simulink library "fixpt_megmalib"  (Simulink 6.0)
settings: Solver=ode45  SolverMode=SingleTasking  StartTime=0.0  StopTime=10.0  RelTol=1e-3
undefined symbols (not defined in the file or in its folder): Bias1, Bias2, NumBits1, NumBits2, Slope1, Slope2
libraries: simulink x94, fixpt_megmaFuncBlkhidden1 x5, fixpt_megmalib x3
(part 2 of 3)

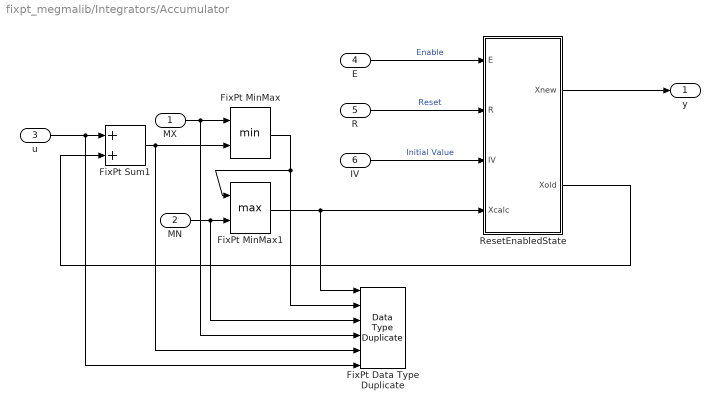
== system fixpt_megmalib/Integrators/Accumulator ==
  MX : Inport  LatchInput=off
  MN : Inport  Port=2  LatchInput=off
  u : Inport  Port=3  LatchInput=off
  E : Inport  Port=4  LatchInput=off
  R : Inport  Port=5  LatchInput=off
  IV : Inport  Port=6  LatchInput=off
  FixPt Data Type Duplicate : simulink/Signal Attributes/Data Type Duplicate  NumInputPorts=6
  FixPt MinMax : MinMax  Inputs=2  OutScaling=2^-10  ZeroCross=off
  FixPt MinMax1 : MinMax  Function=max  Inputs=2  OutScaling=2^-10  ZeroCross=off
  FixPt Sum1 : Sum  OutDataType=uint(4)  OutScaling=1  LockScale=on
  ResetEnabledState : Subsystem  PropExecContextAcrossSSBoundary=on
  y : Outport
  wires:
  ResetEnabledState/2(Xold) -> FixPt Sum1/2
  ResetEnabledState/1(Xnew) -> y/1
  IV/1 -> ResetEnabledState/3(IV)  "Initial Value"
  E/1 -> ResetEnabledState/1(E)  "Enable"
  R/1 -> ResetEnabledState/2(R)  "Reset"
  FixPt MinMax1/1 -> FixPt Data Type Duplicate/1, ResetEnabledState/4(Xcalc)
  MN/1 -> FixPt Data Type Duplicate/3, FixPt MinMax1/2
  FixPt MinMax/1 -> FixPt Data Type Duplicate/2, FixPt MinMax1/1
  MX/1 -> FixPt Data Type Duplicate/4, FixPt MinMax/1
  FixPt Sum1/1 -> FixPt Data Type Duplicate/5, FixPt MinMax/2
  u/1 -> FixPt Data Type Duplicate/6, FixPt Sum1/1

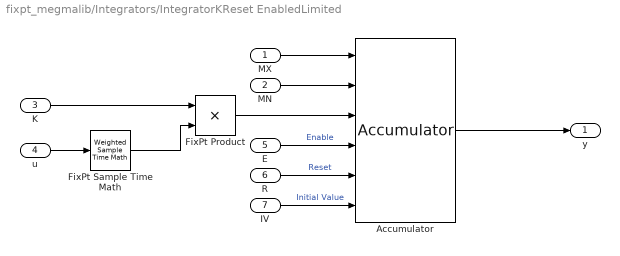
== system fixpt_megmalib/Integrators/IntegratorKReset EnabledLimited ==
  MX : Inport  LatchInput=off
  MN : Inport  Port=2  LatchInput=off
  K : Inport  Port=3  LatchInput=off
  u : Inport  Port=4  LatchInput=off
  E : Inport  Port=5  LatchInput=off
  R : Inport  Port=6  LatchInput=off
  IV : Inport  Port=7  LatchInput=off
  Accumulator : fixpt_megmalib/Integrators/Accumulator
  FixPt Product : Product  OutScaling=2^-10
  FixPt Sample Time Math : simulink/Math Operations/Weighted Sample Time Math  TsampMathOp=*  weightValue=1.0  TsampMathImp=Online Calculations  DoSatur=off
  y : Outport
  wires:
  Accumulator/1 -> y/1
  K/1 -> FixPt Product/1
  FixPt Sample Time Math/1 -> FixPt Product/2
  u/1 -> FixPt Sample Time Math/1
  FixPt Product/1 -> Accumulator/3
  MX/1 -> Accumulator/1
  MN/1 -> Accumulator/2
  R/1 -> Accumulator/5  "Reset"
  E/1 -> Accumulator/4  "Enable"
  IV/1 -> Accumulator/6  "Initial Value"

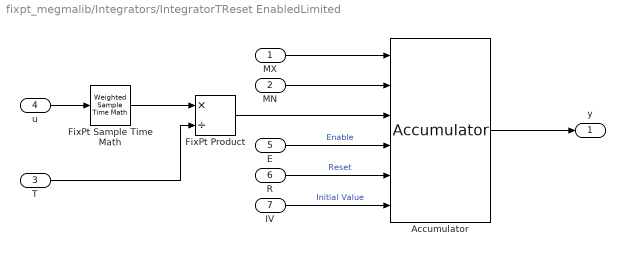
== system fixpt_megmalib/Integrators/IntegratorTReset EnabledLimited ==
  MX : Inport  LatchInput=off
  MN : Inport  Port=2  LatchInput=off
  T : Inport  Port=3  LatchInput=off
  u : Inport  Port=4  LatchInput=off
  E : Inport  Port=5  LatchInput=off
  R : Inport  Port=6  LatchInput=off
  IV : Inport  Port=7  LatchInput=off
  Accumulator : fixpt_megmalib/Integrators/Accumulator
  FixPt Product : Product  Inputs=*/  OutScaling=2^-10
  FixPt Sample Time Math : simulink/Math Operations/Weighted Sample Time Math  TsampMathOp=*  weightValue=1.0  TsampMathImp=Online Calculations  DoSatur=off
  y : Outport
  wires:
  Accumulator/1 -> y/1
  FixPt Product/1 -> Accumulator/3
  MX/1 -> Accumulator/1
  MN/1 -> Accumulator/2
  R/1 -> Accumulator/5  "Reset"
  E/1 -> Accumulator/4  "Enable"
  IV/1 -> Accumulator/6  "Initial Value"
  u/1 -> FixPt Sample Time Math/1
  FixPt Sample Time Math/1 -> FixPt Product/1
  T/1 -> FixPt Product/2

== system fixpt_megmalib/Low and Highpass/DigitalLowPass ResetEnabled ==
  m : Inport  LatchInput=off
  U : Inport  Port=2  LatchInput=off
  E : Inport  Port=3  LatchInput=off
  R : Inport  Port=4  LatchInput=off
  IV : Inport  Port=5  LatchInput=off
  Combine Terms1 : Sum  Description=\nAdd in CPU  OutDataType=sfix(32)  OutScaling=2^-24
  Difference Inputs : Sum  Description=\nAdd in CPU  Inputs=+-  OutDataType=BaseType  OutScaling=1
  FixPt Data Type Duplicate : simulink/Signal Attributes/Data Type Duplicate  NumInputPorts=6
  FixPt Product : Product  OutScaling=2^-10
  ResetEnabledState : Subsystem  PropExecContextAcrossSSBoundary=on
  y : Outport
  wires:
  m/1 -> FixPt Product/1
  Difference Inputs/1 -> FixPt Data Type Duplicate/4, FixPt Product/2
  U/1 -> FixPt Data Type Duplicate/5, Difference Inputs/1  "U(k)"
  ResetEnabledState/2(Xold) -> FixPt Data Type Duplicate/1, Difference Inputs/2, Combine Terms1/2  "Xold"
  ResetEnabledState/1(Xnew) -> y/1  "Xnew"
  E/1 -> ResetEnabledState/1(E)  "Enable"
  IV/1 -> FixPt Data Type Duplicate/6, ResetEnabledState/3(IV)  "Initial Value"
  R/1 -> ResetEnabledState/2(R)  "Reset"
  Combine Terms1/1 -> FixPt Data Type Duplicate/2, ResetEnabledState/4(Xcalc)  "Y(k)"
  FixPt Product/1 -> FixPt Data Type Duplicate/3, Combine Terms1/1

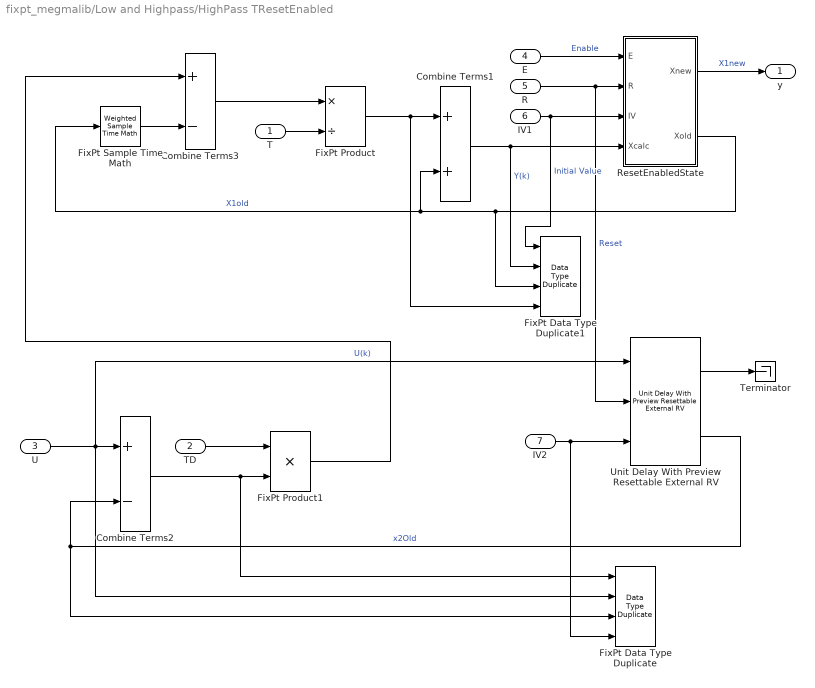
== system fixpt_megmalib/Low and Highpass/HighPass TResetEnabled ==
  T : Inport  LatchInput=off
  TD : Inport  Port=2  LatchInput=off
  U : Inport  Port=3  LatchInput=off
  E : Inport  Port=4  LatchInput=off
  R : Inport  Port=5  LatchInput=off
  IV1 : Inport  Port=6  LatchInput=off
  IV2 : Inport  Port=7  LatchInput=off
  Combine Terms1 : Sum  Description=\nAdd in CPU  OutDataType=sfix(32)  OutScaling=2^-24
  Combine Terms2 : Sum  Description=\nAdd in CPU  Inputs=+-  OutDataType=sfix(32)  OutScaling=2^-24
  Combine Terms3 : Sum  Description=\nAdd in CPU  Inputs=+-  OutDataType=sfix(32)  OutScaling=2^-24
  FixPt Data Type Duplicate : simulink/Signal Attributes/Data Type Duplicate  NumInputPorts=4
  FixPt Data Type Duplicate1 : simulink/Signal Attributes/Data Type Duplicate  NumInputPorts=4
  FixPt Product : Product  Inputs=*/  OutScaling=2^-10
  FixPt Product1 : Product  Inputs=**  OutScaling=2^-10
  FixPt Sample Time Math : simulink/Math Operations/Weighted Sample Time Math  TsampMathOp=*  weightValue=1.0  TsampMathImp=Online Calculations  DoSatur=off
  ResetEnabledState : Subsystem  PropExecContextAcrossSSBoundary=on
  Terminator : Terminator
  Unit Delay With Preview Resettable External RV : simulink/Additional Math & Discrete/Additional Discrete/Unit Delay With Preview Resettable External RV  vinit=0.0  tsamp=-1
  y : Outport
  wires:
  FixPt Product1/1 -> Combine Terms3/1
  FixPt Sample Time Math/1 -> Combine Terms3/2
  Combine Terms3/1 -> FixPt Product/1
  Combine Terms2/1 -> FixPt Data Type Duplicate/1, FixPt Product1/2
  TD/1 -> FixPt Product1/1
  Unit Delay With Preview Resettable External RV/2 -> FixPt Data Type Duplicate/3, Combine Terms2/2  "x2Old"
  ResetEnabledState/2(Xold) -> FixPt Data Type Duplicate1/3, FixPt Sample Time Math/1, Combine Terms1/2  "X1old"
  Combine Terms1/1 -> FixPt Data Type Duplicate1/2, ResetEnabledState/4(Xcalc)  "Y(k)"
  T/1 -> FixPt Product/2
  IV2/1 -> FixPt Data Type Duplicate/4, Unit Delay With Preview Resettable External RV/3
  FixPt Product/1 -> FixPt Data Type Duplicate1/4, Combine Terms1/1
  R/1 -> ResetEnabledState/2(R), Unit Delay With Preview Resettable External RV/2  "Reset"
  IV1/1 -> FixPt Data Type Duplicate1/1, ResetEnabledState/3(IV)  "Initial Value"
  E/1 -> ResetEnabledState/1(E)  "Enable"
  ResetEnabledState/1(Xnew) -> y/1  "X1new"
  U/1 -> FixPt Data Type Duplicate/2, Combine Terms2/1, Unit Delay With Preview Resettable External RV/1  "U(k)"
  Unit Delay With Preview Resettable External RV/1 -> Terminator/1

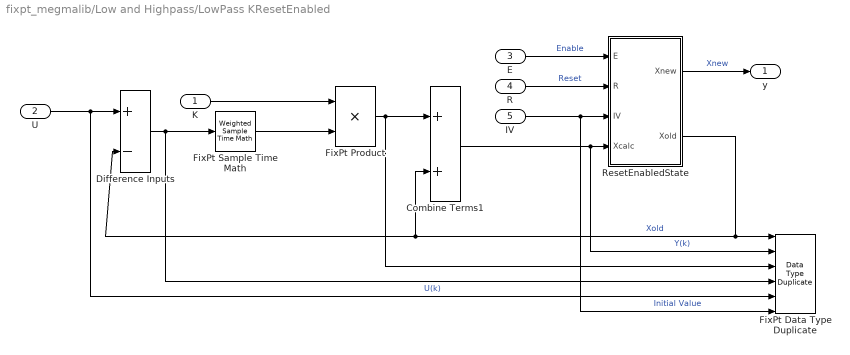
== system fixpt_megmalib/Low and Highpass/LowPass KResetEnabled ==
  K : Inport  LatchInput=off
  U : Inport  Port=2  LatchInput=off
  E : Inport  Port=3  LatchInput=off
  R : Inport  Port=4  LatchInput=off
  IV : Inport  Port=5  LatchInput=off
  Combine Terms1 : Sum  Description=\nAdd in CPU  OutDataType=sfix(32)  OutScaling=2^-24
  Difference Inputs : Sum  Description=\nAdd in CPU  Inputs=+-  OutDataType=BaseType  OutScaling=1
  FixPt Data Type Duplicate : simulink/Signal Attributes/Data Type Duplicate  NumInputPorts=6
  FixPt Product : Product  OutScaling=2^-10
  FixPt Sample Time Math : simulink/Math Operations/Weighted Sample Time Math  TsampMathOp=*  weightValue=1.0  TsampMathImp=Online Calculations  DoSatur=off
  ResetEnabledState : Subsystem  PropExecContextAcrossSSBoundary=on
  y : Outport
  wires:
  FixPt Sample Time Math/1 -> FixPt Product/2
  FixPt Product/1 -> Combine Terms1/1, FixPt Data Type Duplicate/3
  Combine Terms1/1 -> FixPt Data Type Duplicate/2, ResetEnabledState/4(Xcalc)  "Y(k)"
  R/1 -> ResetEnabledState/2(R)  "Reset"
  IV/1 -> FixPt Data Type Duplicate/6, ResetEnabledState/3(IV)  "Initial Value"
  E/1 -> ResetEnabledState/1(E)  "Enable"
  ResetEnabledState/1(Xnew) -> y/1  "Xnew"
  ResetEnabledState/2(Xold) -> Combine Terms1/2, Difference Inputs/2, FixPt Data Type Duplicate/1  "Xold"
  U/1 -> Difference Inputs/1, FixPt Data Type Duplicate/5  "U(k)"
  Difference Inputs/1 -> FixPt Data Type Duplicate/4, FixPt Sample Time Math/1
  K/1 -> FixPt Product/1

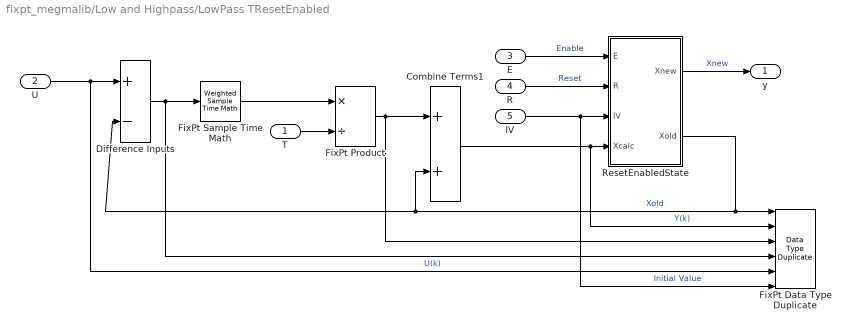
== system fixpt_megmalib/Low and Highpass/LowPass TResetEnabled ==
  T : Inport  LatchInput=off
  U : Inport  Port=2  LatchInput=off
  E : Inport  Port=3  LatchInput=off
  R : Inport  Port=4  LatchInput=off
  IV : Inport  Port=5  LatchInput=off
  Combine Terms1 : Sum  Description=\nAdd in CPU  OutDataType=sfix(32)  OutScaling=2^-24
  Difference Inputs : Sum  Description=\nAdd in CPU  Inputs=+-  OutDataType=BaseType  OutScaling=1
  FixPt Data Type Duplicate : simulink/Signal Attributes/Data Type Duplicate  NumInputPorts=6
  FixPt Product : Product  Inputs=*/  OutScaling=2^-10
  FixPt Sample Time Math : simulink/Math Operations/Weighted Sample Time Math  TsampMathOp=*  weightValue=1.0  TsampMathImp=Online Calculations  DoSatur=off
  ResetEnabledState : Subsystem  PropExecContextAcrossSSBoundary=on
  y : Outport
  wires:
  T/1 -> FixPt Product/2
  Difference Inputs/1 -> FixPt Sample Time Math/1, FixPt Data Type Duplicate/4
  U/1 -> FixPt Data Type Duplicate/5, Difference Inputs/1  "U(k)"
  ResetEnabledState/2(Xold) -> FixPt Data Type Duplicate/1, Difference Inputs/2, Combine Terms1/2  "Xold"
  ResetEnabledState/1(Xnew) -> y/1  "Xnew"
  E/1 -> ResetEnabledState/1(E)  "Enable"
  IV/1 -> FixPt Data Type Duplicate/6, ResetEnabledState/3(IV)  "Initial Value"
  R/1 -> ResetEnabledState/2(R)  "Reset"
  Combine Terms1/1 -> FixPt Data Type Duplicate/2, ResetEnabledState/4(Xcalc)  "Y(k)"
  FixPt Product/1 -> FixPt Data Type Duplicate/3, Combine Terms1/1
  FixPt Sample Time Math/1 -> FixPt Product/1

== system fixpt_megmalib/Mathematical Functions/Configurable Subsystem ==
  In1 : Inport  LatchInput=off
  Sine : fixpt_megmaFuncBlkhidden1/Sine  yData=[1 2 3]  xData=[1 2 3]  Recompute=Compute Always  Spacing='pow2'  Nptsmax=[]  ErrMax=0.01  RndMeth='floor'  yScale=2^-5  xScale=2^-5  yDt=sfix(16)  xDt=sfix(16)  xmax=2*pi  xmin=0
  Out1 : Outport
  wires:
  In1/1 -> Sine/1
  Sine/1 -> Out1/1

== system fixpt_megmalib/Mathematical Functions/Configurable Subsystem1 ==
  In1 : Inport  LatchInput=off
  Cosine : fixpt_megmaFuncBlkhidden1/Cosine  yData=[1 2 3]  xData=[1 2 3]  Recompute=Compute Always  yData_nonvisible=[1;0.999511758485136;0.998047510700099;0.995608686458002;0.992197667229329;0.987817783816472;0.982473313101255;0.976169473868635;0.968912421710645;0.960709243015562;0.951567948048172;0.941497463127881;0.930507621912314;0.918609155794918;0.905813683425936;0.892133699366994;0.877582561890373;0.86217447993488;0.845924499231068;0.828848487609326;0.810963119505218;0.792285859677179;0.772834946152472;0.752629372418066;0.731688868873821;0.71003388356608;0.687685562220505;0.664665727593633;0.640996858163325;0.616702066178912;0.591805075092477;0.566330196393309;0.54030230586814;0.513746819310368;0.486689667701963;0.459157271892304;0.431176516798666;0.402774725153557;0.373979630824533;0.344819351732545;0.315322362395269;0.28551746612222;0.255433766888812;0.225100640916817;0.194547707988987;0.163804802525833;0.132901944452825;0.101869309886441;0.0707372016677029;0.0395360197719658;0.00829623162385838;-0.0229516576536404;-0.0541771350269363;-0.0853497093472792;-0.116438941124852;-0.147414472252418;-0.178246055649492;-0.208903584798109;-0.239357123141322;-0.269576933315742;-0.299533506189574;-0.329197589677777;-0.358540217306233;-0.387532736497014;-0.416146836547142;-0.444354576273508;-0.47212841129696;-0.499441220938929;-0.526266334704305;-0.552577558324725;-0.578349199336833;-0.603556092170533;-0.628173622722739;-0.652177752392634;-0.675545041554953;-0.698252672448376;-0.720278471456692;-0.741600930760952;-0.762199229341495;-0.782053253309314;-0.801143615546934;-0.819451674639598;-0.836959553078294;-0.853650154716842;-0.869507181465984;-0.884515149208199;-0.898659402917676;-0.911926130970699;-0.924302378632464;-0.935776060707157;-0.946335973338945;-0.955971804952348;-0.964674146321316;-0.972434499757186;-0.979245287406521;-0.985099858650763;-0.989992496600445;-0.993918423677641;-0.996873806281181;-0.998855758530109;-0.999862345081687;-0.999892583021229;-0.9989464428219;-0.99702484837355;-0.994129676080546;-0.990263753029502;-0.98543085422867;-0.979635698921714;-0.972883945979446;-0.965182188374036;-0.956537946741083;-0.946959662035847;-0.936456687290796;-0.925039278482532;-0.912718584516998;-0.899506636342767;-0.88541633520302;-0.870461440037704;-0.85465655404816;-0.838017110437342;-0.820559357339561;-0.802300341954454;-0.783257893900684;-0.76345060780562;-0.742897825147999;-0.721619615371299;-0.699636756286272;-0.676970713781757;-0.653643620863612;-0.629678256042204;-0.605098021089583;-0.579926918188046;-0.554189526492417;-0.527910978128915;-0.501116933654064;-0.47383355699759;-0.446087489913793;-0.417905825966321;-0.38931608407177;-0.360346181627922;-0.331024407252887;-0.301379393161745;-0.271440087207671;-0.24123572461485;-0.21079579943078;-0.180150035725827;-0.149328358568183;-0.118360864802541;-0.0872777936610349;-0.0561094972351469;-0.0248864108374021;0.00636097671819611;0.0376021528879766;0.0688066111935807;0.0999438810110212;0.130983557324729;0.161895330417537;0.192649015467599;0.223214582023364;0.253562183327795;0.283662185463226;0.313485196288377;0.343002094139282;0.372184056266098;0.401002586978036;0.429429545468913;0.457437173296176;0.484998121486549;0.512085477241841;0.538672790218836;0.564734098357607;0.590243953233023;0.615177444904708;0.639510226241173;0.663218536694376;0.686279225501496;0.70866977429126;0.730368319072748;0.751353671585211;0.771605339988047;0.791103548870739;0.809829258563201;0.827764183727699;0.844890811214172;0.861192417161521;0.876653083328182;0.891257712636015;0.904992043912346;0.917842665815758;0.929797029932041;0.940843463027505;0.950971178447692;0.960170286650366;0.968431804862477;0.975747665851692;0.982110725803907;0.987514771299061;0.991954525378437;0.995425652697519;0.997924763759387;0.999449418224499;0.999998127293645]  xData_nonvisible=[0;0.03125;0.0625;0.09375;0.125;0.15625;0.1875;0.21875;0.25;0.28125;0.3125;0.34375;0.375;0.40625;0.4375;0.46875;0.5;0.53125;0.5625;0.59375;0.625;0.65625;0.6875;0.71875;0.75;0.78125;0.8125;0.84375;0.875;0.90625;0.9375;0.96875;1;1.03125;1.0625;1.09375;1.125;1.15625;1.1875;1.21875;1.25;1.28125;1.3125;1.34375;1.375;1.40625;1.4375;1.46875;1.5;1.53125;1.5625;1.59375;1.625;1.65625;1.6875;1.71875;1.75;1.78125;1.8125;1.84375;1.875;1.90625;1.9375;1.96875;2;2.03125;2.0625;2.09375;2.125;2.15625;2.1875;2.21875;2.25;2.28125;2.3125;2.34375;2.375;2.40625;2.4375;2.46875;2.5;2.53125;2.5625;2.59375;2.625;2.65625;2.6875;2.71875;2.75;2.78125;2.8125;2.84375;2.875;2.90625;2.9375;2.96875;3;3.03125;3.0625;3.09375;3.125;3.15625;3.1875;3.21875;3.25;3.28125;3.3125;3.34375;3.375;3.40625;3.4375;3.46875;3.5;3.53125;3.5625;3.59375;3.625;3.65625;3.6875;3.71875;3.75;3.78125;3.8125;3.84375;3.875;3.90625;3.9375;3.96875;4;4.03125;4.0625;4.09375;4.125;4.15625;4.1875;4.21875;4.25;4.28125;4.3125;4.34375;4.375;4.40625;4.4375;4.46875;4.5;4.53125;4.5625;4.59375;4.625;4.65625;4.6875;4.71875;4.75;4.78125;4.8125;4.84375;4.875;4.90625;4.9375;4.96875;5;5.03125;5.0625;5.09375;5.125;5.15625;5.1875;5.21875;5.25;5.28125;5.3125;5.34375;5.375;5.40625;5.4375;5.46875;5.5;5.53125;5.5625;5.59375;5.625;5.65625;5.6875;5.71875;5.75;5.78125;5.8125;5.84375;5.875;5.90625;5.9375;5.96875;6;6.03125;6.0625;6.09375;6.125;6.15625;6.1875;6.21875;6.25;6.28125]  Spacing_nonvisible='pow2'  Nptsmax_nonvisible=[]  ErrMax_nonvisible=0.01  RndMeth_nonvisible='floor'  yScale_nonvisible=2^-5  yDt_nonvisible=sfix(16)  xScale_nonvisible=2^-5  xDt_nonvisible=sfix(16)  xMax_nonvisible=2*pi  xMin_nonvisible=0  Spacing='pow2'  Nptsmax=[]  ErrMax=0.01  RndMeth='floor'  yScale=2^-5  xScale=2^-5  yDt=sfix(16)  xDt=sfix(16)  xmax=2*pi  xmin=0
  Out1 : Outport
  wires:
  In1/1 -> Cosine/1
  Cosine/1 -> Out1/1

== system fixpt_megmalib/Mathematical Functions/Configurable Subsystem2 ==
  In1 : Inport  LatchInput=off
  Tangent : fixpt_megmaFuncBlkhidden1/Tangent  yData=[1 2 3]  xData=[1 2 3]  Recompute=Compute Always  Spacing='pow2'  Nptsmax=[]  ErrMax=0.01  RndMeth='floor'  yScale=2^-5  xScale=2^-5  yDt=sfix(16)  xDt=sfix(16)  xmax=2*pi  xmin=0
  Out1 : Outport
  wires:
  In1/1 -> Tangent/1
  Tangent/1 -> Out1/1

== system fixpt_megmalib/Mathematical Functions/Configurable Subsystem3 ==
  In1 : Inport  LatchInput=off
  Exponent : fixpt_megmaFuncBlkhidden1/Exponent  yData=[1 2 3]  xData=[1 2 3]  Recompute=Compute Always  yData_nonvisible=[1;1.0317434074991;1.06449445891786;1.09828514030783;1.13314845306683;1.1691184461695;1.20623024942098;1.2445201077661;1.28402541668774;1.32478475872887;1.3668379411738;1.41022603492571;1.4549914146182;1.50117780000012;1.54883029863413;1.59799544995063;1.64872127070013;1.7010573018484;1.7550546569603;1.81076607211939;1.86824595743222;1.92755045016754;1.98873746958229;2.05186677348798;2.11700001661267;2.18420081081562;2.25353478721321;2.32506966027712;2.3988752939671;2.47502376996303;2.55358945806293;2.63464908881563;2.71828182845905;2.80456935623723;2.89359594417176;2.98544853936536;3.08021684891803;3.17799342753884;3.27887376793867;3.38295639409247;3.49034295746184;3.60113833627218;3.7154507379411;3.83339180475841;3.95507672292058;4.08062433502646;4.21015725614396;4.34380199356104;4.48168907033806;4.62395315278208;4.7707331819676;4.92217250943229;5.07841903718008;5.23962536212849;5.40594892514117;5.57755216479126;5.75460267600573;5.93727337374561;6.12574266188199;6.32019460743274;6.52081912033011;6.72781213889469;6.94137582119704;7.16171874249371;7.38905609893065;7.62360991771274;7.86560927394489;8.11529051435645;8.37289748812726;8.6386817850411;8.91290298119874;9.1958288925309;9.48773583635853;9.78890890125589;10.0996422254801;10.4202392842386;10.7510131860764;11.0922869786702;11.4443939643311;11.8076780255212;12.1824939607035;12.5692078308534;12.9681973169691;13.3798520889305;13.8045741860671;14.242778409807;14.6948927287889;15.1613586968345;15.6426318841882;16.1391823224464;16.6514949636101;17.1800701537093;17.7254241214616;18.2880894824436;18.8686157592649;19.4675699182552;20.0855369231877;20.7231203065787;21.3809427591233;22.0596467378412;22.7598950935267;23.4823717181174;24.227782212611;24.9968545761854;25.7903399171931;26.6090131867249;27.4536739354601;28.3251470945409;29.2242837812349;30.1519621301721;31.1090881509677;32.0965966130693;33.1154519586923;34.166649244734;35.2512151145885;36.3702088008095;37.524723159601;38.7158857381472;39.9448598758219;41.2128458403547;42.5210820000628;43.8708460332935;45.2634561762588;46.7002725104795;48.1826982910988;49.7121813173595;51.2902153465857;52.9183415530491;54.5981500331442;56.3312813583435;58.119428177448;59.9643368696996;61.8678092503679;63.8317043304791;65.8579401324037;67.9484955630781;70.1054123466879;72.3307970187014;74.6268229832009;76.9957326355201;79.4398395522613;81.9615307508321;84.563269020706;87.2475953286865;90.0171313005218;92.8745817812945;95.8227374770869;98.8644776805016;102.0027730827;105.240688674702;108.58138674079;112.02812994692;115.584284527188;119.253323571426;123.038830417177;126.944502149322;130.974153210819;135.13171912804;139.421260354375;143.846966235843;148.413159102577;153.124298490199;157.984985495187;162.999967268501;168.174141651845;173.512561961112;179.020441921657;184.703160760245;190.56626845863;196.615491173896;202.856736830865;209.296100892025;215.939872310614;222.794539672674;229.866797534079;237.163552958717;244.69193226422;252.459287981826;260.473206037167;268.741513159002;277.272284523134;286.073851638959;295.154810486372;304.524029910962;314.190660285694;324.164142447555;334.454216917865;345.070933415282;356.024660670779;367.326096554181;378.986278522156;391.016594397853;403.428793492735;416.234998081446;429.447715240934;443.079849065385;457.144713268909;471.656044188264;486.628014198347;502.075245553524;518.012824668342;534.45631685155]  xData_nonvisible=[0;0.03125;0.0625;0.09375;0.125;0.15625;0.1875;0.21875;0.25;0.28125;0.3125;0.34375;0.375;0.40625;0.4375;0.46875;0.5;0.53125;0.5625;0.59375;0.625;0.65625;0.6875;0.71875;0.75;0.78125;0.8125;0.84375;0.875;0.90625;0.9375;0.96875;1;1.03125;1.0625;1.09375;1.125;1.15625;1.1875;1.21875;1.25;1.28125;1.3125;1.34375;1.375;1.40625;1.4375;1.46875;1.5;1.53125;1.5625;1.59375;1.625;1.65625;1.6875;1.71875;1.75;1.78125;1.8125;1.84375;1.875;1.90625;1.9375;1.96875;2;2.03125;2.0625;2.09375;2.125;2.15625;2.1875;2.21875;2.25;2.28125;2.3125;2.34375;2.375;2.40625;2.4375;2.46875;2.5;2.53125;2.5625;2.59375;2.625;2.65625;2.6875;2.71875;2.75;2.78125;2.8125;2.84375;2.875;2.90625;2.9375;2.96875;3;3.03125;3.0625;3.09375;3.125;3.15625;3.1875;3.21875;3.25;3.28125;3.3125;3.34375;3.375;3.40625;3.4375;3.46875;3.5;3.53125;3.5625;3.59375;3.625;3.65625;3.6875;3.71875;3.75;3.78125;3.8125;3.84375;3.875;3.90625;3.9375;3.96875;4;4.03125;4.0625;4.09375;4.125;4.15625;4.1875;4.21875;4.25;4.28125;4.3125;4.34375;4.375;4.40625;4.4375;4.46875;4.5;4.53125;4.5625;4.59375;4.625;4.65625;4.6875;4.71875;4.75;4.78125;4.8125;4.84375;4.875;4.90625;4.9375;4.96875;5;5.03125;5.0625;5.09375;5.125;5.15625;5.1875;5.21875;5.25;5.28125;5.3125;5.34375;5.375;5.40625;5.4375;5.46875;5.5;5.53125;5.5625;5.59375;5.625;5.65625;5.6875;5.71875;5.75;5.78125;5.8125;5.84375;5.875;5.90625;5.9375;5.96875;6;6.03125;6.0625;6.09375;6.125;6.15625;6.1875;6.21875;6.25;6.28125]  Spacing_nonvisible='pow2'  Nptsmax_nonvisible=[]  ErrMax_nonvisible=0.01  RndMeth_nonvisible='floor'  yScale_nonvisible=2^-5  yDt_nonvisible=sfix(16)  xScale_nonvisible=2^-5  xDt_nonvisible=sfix(16)  xMax_nonvisible=2*pi  xMin_nonvisible=0  Spacing='pow2'  Nptsmax=[]  ErrMax=0.01  RndMeth='floor'  yScale=2^-5  xScale=2^-5  yDt=sfix(16)  xDt=sfix(16)  xmax=2*pi  xmin=0
  Out1 : Outport
  wires:
  In1/1 -> Exponent/1
  Exponent/1 -> Out1/1

== system fixpt_megmalib/Mathematical Functions/Configurable Subsystem4 ==
  In1 : Inport  LatchInput=off
  Sqrt : fixpt_megmaFuncBlkhidden1/Sqrt  yData=[1 2 3]  xData=[1 2 3]  Recompute=Compute Always  Spacing='pow2'  Nptsmax=[]  ErrMax=0.01  RndMeth='floor'  yScale=2^-5  xScale=2^-5  yDt=sfix(16)  xDt=sfix(16)  xmax=2*pi  xmin=0
  Out1 : Outport
  wires:
  In1/1 -> Sqrt/1
  Sqrt/1 -> Out1/1

== system fixpt_megmalib/Memory Blocks/DeltaOneStep ==
  note: IV
  U : Inport  LatchInput=off
  R : Inport  Port=2  LatchInput=off
  R1 : Inport  Port=3  LatchInput=off
  Data Type Duplicate : simulink/Signal Attributes/Data Type Duplicate  NumInputPorts=4
  Delay Input1 : UnitDelay  Description=\nStore in Global RAM  SampleTime=-1
  Difference Inputs1 : Sum  Description=\nAdd in CPU  Inputs=+-  OutDataType=BaseType  OutScaling=1
  Switch : Switch  Criteria=u2 ~= 0
  Y : Outport  InitialOutput=0
  wires:
  U/1 -> Data Type Duplicate/2, Difference Inputs1/1, Delay Input1/1  "U(k)"
  R/1 -> Switch/2
  R1/1 -> Data Type Duplicate/4, Switch/1
  Delay Input1/1 -> Switch/3  "U(k-1)"
  Difference Inputs1/1 -> Data Type Duplicate/1, Y/1  "( U(k) - U(k-1) )"
  Switch/1 -> Data Type Duplicate/3, Difference Inputs1/2

== system fixpt_megmalib/Memory Blocks/DifferenceQuotient ==
  u : Inport  LatchInput=off
  R : Inport  Port=2  LatchInput=off
  IV : Inport  Port=3  LatchInput=off
  DeltaOneStep : fixpt_megmalib/Memory Blocks/DeltaOneStep
  Sample Time Divide : simulink/Math Operations/Weighted Sample Time Math  TsampMathOp=/  weightValue=1  TsampMathImp=Online Calculations  DoSatur=off
  Y : Outport  InitialOutput=0
  wires:
  Sample Time Divide/1 -> Y/1
  DeltaOneStep/1 -> Sample Time Divide/1
  u/1 -> DeltaOneStep/1
  R/1 -> DeltaOneStep/2
  IV/1 -> DeltaOneStep/3

== system fixpt_megmalib/Memory Blocks/EdgeBi ==
  note: x
  U(k) : Inport  LatchInput=off
  R : Inport  Port=2  LatchInput=off
  IV : Inport  Port=3  LatchInput=off
  Data Type Duplicate : simulink/Signal Attributes/Data Type Duplicate  NumInputPorts=3
  Delay Input1 : UnitDelay  Description=\nStore in Global RAM  SampleTime=-1
  FixPt Relational Operator : RelationalOperator  Operator=~=  LogicOutDataTypeMode=Specify via dialog
  Switch : Switch  Criteria=u2 ~= 0
  Y : Outport  InitialOutput=0
  wires:
  U(k)/1 -> Delay Input1/1, FixPt Relational Operator/1
  FixPt Relational Operator/1 -> Y/1  "Edge"
  R/1 -> Switch/2
  IV/1 -> Data Type Duplicate/2, Switch/1
  Delay Input1/1 -> Data Type Duplicate/3, Switch/3  "U(k-1)"
  Switch/1 -> Data Type Duplicate/1, FixPt Relational Operator/2

== system fixpt_megmalib/Memory Blocks/EdgeFalling ==
  note: x
  U(k) : Inport  LatchInput=off
  R : Inport  Port=2  LatchInput=off
  IV : Inport  Port=3  LatchInput=off
  Data Type Duplicate : simulink/Signal Attributes/Data Type Duplicate  NumInputPorts=3
  Delay Input1 : UnitDelay  Description=\nStore in Global RAM  SampleTime=-1
  Logical Operator : Logic  Operator=NOT  Inputs=1  AllPortsSameDT=off  OutDataTypeMode=Specify via dialog
  Logical Operator1 : Logic  AllPortsSameDT=off  OutDataTypeMode=Specify via dialog
  Switch : Switch  Criteria=u2 ~= 0
  Y : Outport  InitialOutput=0
  wires:
  Delay Input1/1 -> Data Type Duplicate/2, Switch/3  "U(k-1)"
  IV/1 -> Data Type Duplicate/3, Switch/1
  R/1 -> Switch/2
  Logical Operator1/1 -> Y/1  "Edge"
  U(k)/1 -> Delay Input1/1, Logical Operator/1
  Switch/1 -> Data Type Duplicate/1, Logical Operator1/2
  Logical Operator/1 -> Logical Operator1/1

== system fixpt_megmalib/Memory Blocks/EdgeRising ==
  note: x
  U(k) : Inport  LatchInput=off
  R : Inport  Port=2  LatchInput=off
  IV : Inport  Port=3  LatchInput=off
  Data Type Duplicate : simulink/Signal Attributes/Data Type Duplicate  NumInputPorts=3
  Delay Input1 : UnitDelay  Description=\nStore in Global RAM  SampleTime=-1
  Logical Operator : Logic  Operator=NOT  Inputs=1  AllPortsSameDT=off  OutDataTypeMode=Specify via dialog
  Logical Operator1 : Logic  AllPortsSameDT=off  OutDataTypeMode=Specify via dialog
  Switch : Switch  Criteria=u2 ~= 0
  Y : Outport  InitialOutput=0
  wires:
  U(k)/1 -> Delay Input1/1, Logical Operator1/1
  Logical Operator1/1 -> Y/1  "Edge"
  R/1 -> Switch/2
  IV/1 -> Data Type Duplicate/2, Switch/1
  Delay Input1/1 -> Data Type Duplicate/3, Switch/3  "U(k-1)"
  Switch/1 -> Data Type Duplicate/1, Logical Operator/1
  Logical Operator/1 -> Logical Operator1/2

== system fixpt_megmalib/Memory Blocks/RSFlipFlop ==
  S : Inport  LatchInput=off
  R : Inport  Port=2  LatchInput=off
  Constant : Constant  OutDataTypeMode=boolean
  FixPt Data Type Duplicate1 : simulink/Signal Attributes/Data Type Duplicate  NumInputPorts=5
  FixPt Switch1 : Switch  Threshold=1
  FixPt Switch3 : Switch  Threshold=1
  FixPt Unit Delay1 : UnitDelay  X0=0.0  SampleTime=-1
  Ground : Ground
  Logical Operator : Logic  Operator=NOT  Inputs=1  AllPortsSameDT=off
  Q : Outport  InitialOutput=0
  !Q : Outport  Port=2  InitialOutput=1
  wires:
  Logical Operator/1 -> !Q/1
  Ground/1 -> FixPt Data Type Duplicate1/3, FixPt Switch1/1
  Constant/1 -> FixPt Data Type Duplicate1/5, FixPt Switch3/1
  S/1 -> FixPt Switch3/2  "Set"
  FixPt Switch3/1 -> FixPt Data Type Duplicate1/4, FixPt Switch1/3
  FixPt Unit Delay1/1 -> FixPt Switch3/3, FixPt Data Type Duplicate1/1  "Xold"
  FixPt Switch1/1 -> Logical Operator/1, Q/1, FixPt Data Type Duplicate1/2, FixPt Unit Delay1/1  "Xnew"
  R/1 -> FixPt Switch1/2  "Reset"

== system fixpt_megmalib/Memory Blocks/SampleAndHold ResetEnabled ==
  note: x
  note: x
  U(k) : Inport  LatchInput=off
  R : Inport  Port=2  LatchInput=off
  IV : Inport  Port=3  LatchInput=off
  E : Inport  Port=4  LatchInput=off
  Data Type Duplicate : simulink/Signal Attributes/Data Type Duplicate  NumInputPorts=4
  Switch : Switch  Criteria=u2 ~= 0
  Switch1 : Switch  Criteria=u2 ~= 0
  Unit Delay : UnitDelay  Orientation=left  X0=0.0  SampleTime=-1
  Y : Outport  InitialOutput=0
  wires:
  Unit Delay/1 -> Switch/3
  R/1 -> Switch1/2
  IV/1 -> Data Type Duplicate/2, Switch1/1
  E/1 -> Switch/2
  Switch/1 -> Data Type Duplicate/3, Switch1/3
  Switch1/1 -> Data Type Duplicate/1, Unit Delay/1, Y/1
  U(k)/1 -> Data Type Duplicate/4, Switch/1

== system fixpt_megmalib/Nonlinear Blocks/DeadBand ==
  UMAX : Inport  LatchInput=off
  UMIN : Inport  Port=2  LatchInput=off
  u : Inport  Port=3  LatchInput=off
  Dead Zone Dynamic : simulink/Discontinuities/Dead Zone Dynamic
  y : Outport
  wires:
  UMAX/1 -> Dead Zone Dynamic/1
  u/1 -> Dead Zone Dynamic/2
  UMIN/1 -> Dead Zone Dynamic/3
  Dead Zone Dynamic/1 -> y/1

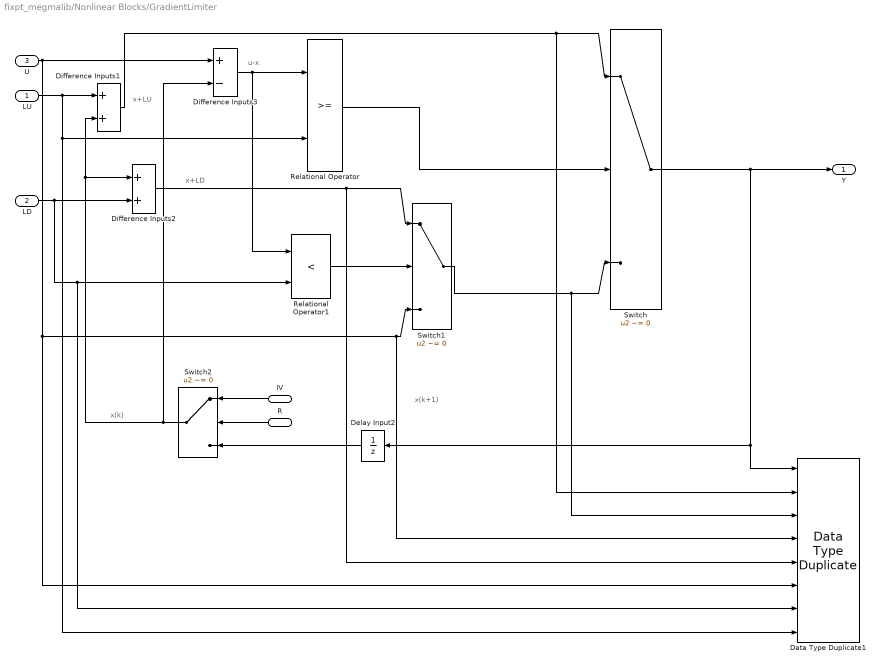
== system fixpt_megmalib/Nonlinear Blocks/GradientLimiter ==
  note: x+LD
  note: x+LU
  note: u-x
  note: x(k+1)
  note: x(k)
  LU : Inport  LatchInput=off
  LD : Inport  Port=2  LatchInput=off
  U : Inport  Port=3  LatchInput=off
  R : Inport  Orientation=left  Port=4  LatchInput=off
  IV : Inport  Orientation=left  Port=5  LatchInput=off
  Data Type Duplicate1 : simulink/Signal Attributes/Data Type Duplicate  NumInputPorts=8
  Delay Input2 : UnitDelay  Description=\nStore in Global RAM  Orientation=left
  Difference Inputs1 : Sum  Description=\nAdd in CPU  OutDataType=BaseType  OutScaling=1
  Difference Inputs2 : Sum  Description=\nAdd in CPU  OutDataType=BaseType  OutScaling=1
  Difference Inputs3 : Sum  Description=\nAdd in CPU  Inputs=+-  OutDataType=BaseType  OutScaling=1
  Relational Operator : RelationalOperator  LogicOutDataTypeMode=Specify via dialog  ZeroCross=off
  Relational Operator1 : RelationalOperator  Operator=<  LogicOutDataTypeMode=Specify via dialog  ZeroCross=off
  Switch : Switch  Criteria=u2 ~= 0  ZeroCross=off
  Switch1 : Switch  Criteria=u2 ~= 0  ZeroCross=off
  Switch2 : Switch  Orientation=left  Criteria=u2 ~= 0  ZeroCross=off
  Y : Outport  InitialOutput=0
  wires:
  Switch1/1 -> Switch/3, Data Type Duplicate1/3
  Difference Inputs2/1 -> Switch1/1, Data Type Duplicate1/5
  Relational Operator1/1 -> Switch1/2
  Difference Inputs1/1 -> Switch/1, Data Type Duplicate1/2
  Relational Operator/1 -> Switch/2
  Difference Inputs3/1 -> Relational Operator1/1, Relational Operator/1
  Switch/1 -> Y/1, Delay Input2/1, Data Type Duplicate1/1
  U/1 -> Difference Inputs3/1, Switch1/3, Data Type Duplicate1/4, Data Type Duplicate1/6
  LD/1 -> Relational Operator1/2, Data Type Duplicate1/7, Difference Inputs2/2
  LU/1 -> Difference Inputs1/1, Relational Operator/2, Data Type Duplicate1/8
  R/1 -> Switch2/2
  IV/1 -> Switch2/1
  Delay Input2/1 -> Switch2/3
  Switch2/1 -> Difference Inputs1/2, Difference Inputs2/1, Difference Inputs3/2

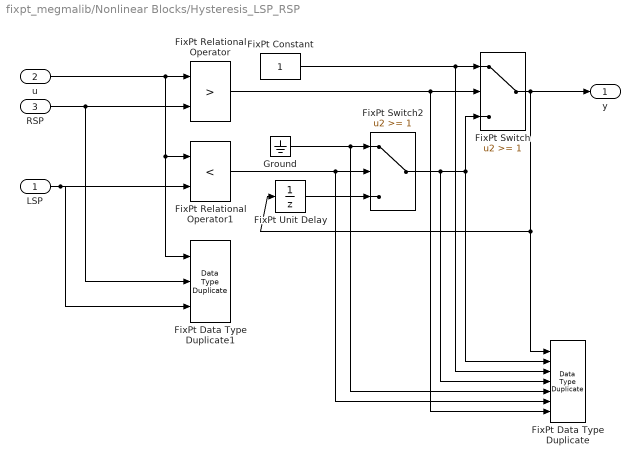
== system fixpt_megmalib/Nonlinear Blocks/Hysteresis_LSP_RSP ==
  LSP : Inport  LatchInput=off
  u : Inport  Port=2  LatchInput=off
  RSP : Inport  Port=3  LatchInput=off
  FixPt Constant : Constant  ConRadixGroup=Best Precision: Vector-wise  OutScaling=2^-14
  FixPt Data Type Duplicate : simulink/Signal Attributes/Data Type Duplicate  NumInputPorts=7
  FixPt Data Type Duplicate1 : simulink/Signal Attributes/Data Type Duplicate  NumInputPorts=3
  FixPt Relational Operator : RelationalOperator  Operator=>  LogicOutDataTypeMode=Specify via dialog  ZeroCross=off
  FixPt Relational Operator1 : RelationalOperator  Operator=<  LogicOutDataTypeMode=Specify via dialog  ZeroCross=off
  FixPt Switch : Switch  Threshold=1  ZeroCross=off
  FixPt Switch2 : Switch  Threshold=1  ZeroCross=off
  FixPt Unit Delay : UnitDelay  X0=0.0  SampleTime=-1
  Ground : Ground
  y : Outport
  wires:
  FixPt Switch/1 -> FixPt Data Type Duplicate/1, FixPt Unit Delay/1, y/1
  FixPt Unit Delay/1 -> FixPt Switch2/3
  Ground/1 -> FixPt Data Type Duplicate/5, FixPt Switch2/1
  FixPt Relational Operator1/1 -> FixPt Data Type Duplicate/6, FixPt Switch2/2
  FixPt Switch2/1 -> FixPt Data Type Duplicate/4, FixPt Data Type Duplicate/2, FixPt Switch/3
  FixPt Constant/1 -> FixPt Data Type Duplicate/3, FixPt Switch/1
  FixPt Relational Operator/1 -> FixPt Data Type Duplicate/7, FixPt Switch/2
  LSP/1 -> FixPt Relational Operator1/2, FixPt Data Type Duplicate1/3
  RSP/1 -> FixPt Relational Operator/2, FixPt Data Type Duplicate1/2
  u/1 -> FixPt Data Type Duplicate1/1, FixPt Relational Operator1/1, FixPt Relational Operator/1

== system fixpt_megmalib/Nonlinear Blocks/Limiter ==
  MX : Inport  LatchInput=off
  MN : Inport  Port=2  LatchInput=off
  u : Inport  Port=3  LatchInput=off
  Saturation Dynamic : simulink/Discontinuities/Saturation Dynamic
  y : Outport
  wires:
  MX/1 -> Saturation Dynamic/1
  MN/1 -> Saturation Dynamic/3
  u/1 -> Saturation Dynamic/2
  Saturation Dynamic/1 -> y/1

== system fixpt_megmalib/Nonlinear Blocks/MaxLogResetEnabled ==
  u : Inport  LatchInput=off
  E : Inport  Port=2  LatchInput=off
  R : Inport  Port=3  LatchInput=off
  IV : Inport  Port=4  LatchInput=off
  Data Type Duplicate : simulink/Signal Attributes/Data Type Duplicate  NumInputPorts=3
  MinMax : MinMax  Function=max  Inputs=2  OutDataType=uint(8)  OutScaling=1  ZeroCross=off
      settings: LockScale=on
  Unit Delay With Preview Enabled Resettable External RV : simulink/Additional Math & Discrete/Additional Discrete/Unit Delay With Preview Enabled Resettable External RV  vinit=0.0  tsamp=-1
  y : Outport
  wires:
  Unit Delay With Preview Enabled Resettable External RV/1 -> y/1
  u/1 -> Data Type Duplicate/3, MinMax/1
  E/1 -> Unit Delay With Preview Enabled Resettable External RV/2  "Enable"
  R/1 -> Unit Delay With Preview Enabled Resettable External RV/3  "Reset"
  IV/1 -> Unit Delay With Preview Enabled Resettable External RV/4  "Initial Value"
  Unit Delay With Preview Enabled Resettable External RV/2 -> Data Type Duplicate/2, MinMax/2
  MinMax/1 -> Unit Delay With Preview Enabled Resettable External RV/1, Data Type Duplicate/1

== system fixpt_megmalib/Nonlinear Blocks/MeanValue ==
  u : Inport  LatchInput=off
  E : Inport  Port=2  LatchInput=off
  R : Inport  Port=3  LatchInput=off
  IV : Inport  Port=4  LatchInput=off
  FixPt Data Type Duplicate : simulink/Signal Attributes/Data Type Duplicate  NumInputPorts=3
  FixPt Data Type Propagation : simulink/Signal Attributes/Data Type Propagation  PropDataType=sfix(16)  IfRefDouble=double  IfRefSingle=single  IsSigned=IsSigned1  NumBitsBase=NumBits1  NumBitsMult=2  NumBitsAdd=0  NumBitsAllowFinal=1:128  PropScaling=2^-10  ValuesUsedBestPrec=[5 -7]  SlopeBase=Slope1  SlopeMult=1  SlopeAdd=0  BiasBase=Bias1+Bias2  BiasMult=1  BiasAdd=0
  FixPt Gain : Gain  Gain=1/nSample  ParameterDataType=ufix(8)  ParameterScalingMode=Use specified scaling  ParameterScaling=2^-1  OutScaling=2^-10
  FixPt Sum : Sum  Inputs=+  OutScaling=2^-10
  ResetEnabledTappedDelay : Subsystem  PropExecContextAcrossSSBoundary=on
      mask Type: Fixed-Point Reset Enabled State
      mask Description:
      | Resetable Enabled State
      | Output
      |   If R % Reset
      |      Xnew = IV
      |   elseif E % Enabled
      |      Xnew = Xen
      |   else
      |      Xnew = Xold % Stays the same
      |   end
      | Update
      |     Xold = Xnew
      mask Display: fprintf('Tapped Delay');
  Y : Outport  InitialOutput=0
  wires:
  E/1 -> ResetEnabledTappedDelay/1(E)
  R/1 -> ResetEnabledTappedDelay/2(R)
  IV/1 -> ResetEnabledTappedDelay/3(IV)
  ResetEnabledTappedDelay/1(Xnew) -> FixPt Data Type Duplicate/2, FixPt Sum/1
  FixPt Sum/1 -> FixPt Data Type Propagation/3, FixPt Gain/1
  u/1 -> FixPt Data Type Duplicate/3, ResetEnabledTappedDelay/4(u), FixPt Data Type Propagation/2, FixPt Data Type Propagation/1
  FixPt Gain/1 -> FixPt Data Type Duplicate/1, Y/1

== system fixpt_megmalib/Nonlinear Blocks/MinLogResetEnabled ==
  u : Inport  LatchInput=off
  E : Inport  Port=2  LatchInput=off
  R : Inport  Port=3  LatchInput=off
  IV : Inport  Port=4  LatchInput=off
  Data Type Duplicate : simulink/Signal Attributes/Data Type Duplicate  NumInputPorts=3
  MinMax : MinMax  Inputs=2  OutDataType=uint(8)  OutScaling=1  ZeroCross=off
      settings: LockScale=on
  Unit Delay With Preview Enabled Resettable External RV : simulink/Additional Math & Discrete/Additional Discrete/Unit Delay With Preview Enabled Resettable External RV  vinit=0.0  tsamp=-1
  y : Outport
  wires:
  Unit Delay With Preview Enabled Resettable External RV/1 -> y/1
  u/1 -> MinMax/1, Data Type Duplicate/3
  E/1 -> Unit Delay With Preview Enabled Resettable External RV/2  "Enable"
  R/1 -> Unit Delay With Preview Enabled Resettable External RV/3  "Reset"
  IV/1 -> Unit Delay With Preview Enabled Resettable External RV/4  "Initial Value"
  Unit Delay With Preview Enabled Resettable External RV/2 -> MinMax/2, Data Type Duplicate/2
  MinMax/1 -> Data Type Duplicate/1, Unit Delay With Preview Enabled Resettable External RV/1

== system fixpt_megmalib/Counters and Timers/CountDown ResetEnabled/ResetEnabledState ==
  E : Inport  LatchInput=off
  R : Inport  Port=2  LatchInput=off
  IV : Inport  Port=3  LatchInput=off
  Xcalc : Inport  Port=4  LatchInput=off
  Unit Delay With Preview Enabled Resettable External RV : simulink/Additional Math & Discrete/Additional Discrete/Unit Delay With Preview Enabled Resettable External RV  vinit=0.0  tsamp=-1
  Xnew : Outport
  Xold : Outport  Port=2
  wires:
  Unit Delay With Preview Enabled Resettable External RV/2 -> Xold/1
  Unit Delay With Preview Enabled Resettable External RV/1 -> Xnew/1
  IV/1 -> Unit Delay With Preview Enabled Resettable External RV/4
  R/1 -> Unit Delay With Preview Enabled Resettable External RV/3
  E/1 -> Unit Delay With Preview Enabled Resettable External RV/2
  Xcalc/1 -> Unit Delay With Preview Enabled Resettable External RV/1

== system fixpt_megmalib/Counters and Timers/CountDown ResetTriggerEnabled/ResetEnabledState ==
  E : Inport  LatchInput=off
  R : Inport  Port=2  LatchInput=off
  IV : Inport  Port=3  LatchInput=off
  Xcalc : Inport  Port=4  LatchInput=off
  Unit Delay With Preview Enabled Resettable External RV : simulink/Additional Math & Discrete/Additional Discrete/Unit Delay With Preview Enabled Resettable External RV  vinit=0.0  tsamp=-1
  Xnew : Outport
  Xold : Outport  Port=2
  wires:
  Unit Delay With Preview Enabled Resettable External RV/2 -> Xold/1
  Unit Delay With Preview Enabled Resettable External RV/1 -> Xnew/1
  IV/1 -> Unit Delay With Preview Enabled Resettable External RV/4
  R/1 -> Unit Delay With Preview Enabled Resettable External RV/3
  E/1 -> Unit Delay With Preview Enabled Resettable External RV/2
  Xcalc/1 -> Unit Delay With Preview Enabled Resettable External RV/1

== system fixpt_megmalib/Counters and Timers/Counter ResetEnabled/ResetEnabledState ==
  E : Inport  LatchInput=off
  R : Inport  Port=2  LatchInput=off
  IV : Inport  Port=3  LatchInput=off
  Xcalc : Inport  Port=4  LatchInput=off
  Unit Delay With Preview Enabled Resettable External RV : simulink/Additional Math & Discrete/Additional Discrete/Unit Delay With Preview Enabled Resettable External RV  vinit=0.0  tsamp=-1
  Xnew : Outport
  Xold : Outport  Port=2
  wires:
  Unit Delay With Preview Enabled Resettable External RV/2 -> Xold/1
  Unit Delay With Preview Enabled Resettable External RV/1 -> Xnew/1
  IV/1 -> Unit Delay With Preview Enabled Resettable External RV/4
  R/1 -> Unit Delay With Preview Enabled Resettable External RV/3
  E/1 -> Unit Delay With Preview Enabled Resettable External RV/2
  Xcalc/1 -> Unit Delay With Preview Enabled Resettable External RV/1

== system fixpt_megmalib/Counters and Timers/Counter ResetTriggerEnabled/ResetEnabledState ==
  E : Inport  LatchInput=off
  R : Inport  Port=2  LatchInput=off
  IV : Inport  Port=3  LatchInput=off
  Xcalc : Inport  Port=4  LatchInput=off
  Unit Delay With Preview Enabled Resettable External RV : simulink/Additional Math & Discrete/Additional Discrete/Unit Delay With Preview Enabled Resettable External RV  vinit=0.0  tsamp=-1
  Xnew : Outport
  Xold : Outport  Port=2
  wires:
  Unit Delay With Preview Enabled Resettable External RV/2 -> Xold/1
  Unit Delay With Preview Enabled Resettable External RV/1 -> Xnew/1
  IV/1 -> Unit Delay With Preview Enabled Resettable External RV/4
  R/1 -> Unit Delay With Preview Enabled Resettable External RV/3
  E/1 -> Unit Delay With Preview Enabled Resettable External RV/2
  Xcalc/1 -> Unit Delay With Preview Enabled Resettable External RV/1

== system fixpt_megmalib/Counters and Timers/StopWatch ResetEnabled/ResetEnabledState ==
  E : Inport  LatchInput=off
  R : Inport  Port=2  LatchInput=off
  IV : Inport  Port=3  LatchInput=off
  Xcalc : Inport  Port=4  LatchInput=off
  Unit Delay With Preview Enabled Resettable External RV : simulink/Additional Math & Discrete/Additional Discrete/Unit Delay With Preview Enabled Resettable External RV  vinit=0.0  tsamp=-1
  Xnew : Outport
  Xold : Outport  Port=2
  wires:
  Unit Delay With Preview Enabled Resettable External RV/2 -> Xold/1
  Unit Delay With Preview Enabled Resettable External RV/1 -> Xnew/1
  IV/1 -> Unit Delay With Preview Enabled Resettable External RV/4
  R/1 -> Unit Delay With Preview Enabled Resettable External RV/3
  E/1 -> Unit Delay With Preview Enabled Resettable External RV/2
  Xcalc/1 -> Unit Delay With Preview Enabled Resettable External RV/1

== system fixpt_megmalib/Counters and Timers/StopWatch ResetTriggerEnabled/ResetEnabledState ==
  E : Inport  LatchInput=off
  R : Inport  Port=2  LatchInput=off
  IV : Inport  Port=3  LatchInput=off
  Xcalc : Inport  Port=4  LatchInput=off
  Unit Delay With Preview Enabled Resettable External RV : simulink/Additional Math & Discrete/Additional Discrete/Unit Delay With Preview Enabled Resettable External RV  vinit=0.0  tsamp=-1
  Xnew : Outport
  Xold : Outport  Port=2
  wires:
  Unit Delay With Preview Enabled Resettable External RV/2 -> Xold/1
  Unit Delay With Preview Enabled Resettable External RV/1 -> Xnew/1
  IV/1 -> Unit Delay With Preview Enabled Resettable External RV/4
  R/1 -> Unit Delay With Preview Enabled Resettable External RV/3
  E/1 -> Unit Delay With Preview Enabled Resettable External RV/2
  Xcalc/1 -> Unit Delay With Preview Enabled Resettable External RV/1

== system fixpt_megmalib/Counters and Timers/Timer ResetEnabled/ResetEnabledState ==
  E : Inport  LatchInput=off
  R : Inport  Port=2  LatchInput=off
  IV : Inport  Port=3  LatchInput=off
  Xcalc : Inport  Port=4  LatchInput=off
  Unit Delay With Preview Enabled Resettable External RV : simulink/Additional Math & Discrete/Additional Discrete/Unit Delay With Preview Enabled Resettable External RV  vinit=0.0  tsamp=-1
  Xnew : Outport
  Xold : Outport  Port=2
  wires:
  Unit Delay With Preview Enabled Resettable External RV/2 -> Xold/1
  Unit Delay With Preview Enabled Resettable External RV/1 -> Xnew/1
  IV/1 -> Unit Delay With Preview Enabled Resettable External RV/4
  R/1 -> Unit Delay With Preview Enabled Resettable External RV/3
  E/1 -> Unit Delay With Preview Enabled Resettable External RV/2
  Xcalc/1 -> Unit Delay With Preview Enabled Resettable External RV/1

== system fixpt_megmalib/Counters and Timers/Timer ResetTriggerEnabled/ResetEnabledState ==
  E : Inport  LatchInput=off
  R : Inport  Port=2  LatchInput=off
  IV : Inport  Port=3  LatchInput=off
  Xcalc : Inport  Port=4  LatchInput=off
  Unit Delay With Preview Enabled Resettable External RV : simulink/Additional Math & Discrete/Additional Discrete/Unit Delay With Preview Enabled Resettable External RV  vinit=0.0  tsamp=-1
  Xnew : Outport
  Xold : Outport  Port=2
  wires:
  Unit Delay With Preview Enabled Resettable External RV/2 -> Xold/1
  Unit Delay With Preview Enabled Resettable External RV/1 -> Xnew/1
  IV/1 -> Unit Delay With Preview Enabled Resettable External RV/4
  R/1 -> Unit Delay With Preview Enabled Resettable External RV/3
  E/1 -> Unit Delay With Preview Enabled Resettable External RV/2
  Xcalc/1 -> Unit Delay With Preview Enabled Resettable External RV/1

== system fixpt_megmalib/Counters and Timers/Timer RetriggerReset TriggerEnabled/ResetEnabledState ==
  E : Inport  LatchInput=off
  R : Inport  Port=2  LatchInput=off
  IV : Inport  Port=3  LatchInput=off
  Xcalc : Inport  Port=4  LatchInput=off
  Unit Delay With Preview Enabled Resettable External RV : simulink/Additional Math & Discrete/Additional Discrete/Unit Delay With Preview Enabled Resettable External RV  vinit=0.0  tsamp=-1
  Xnew : Outport
  Xold : Outport  Port=2
  wires:
  Unit Delay With Preview Enabled Resettable External RV/2 -> Xold/1
  Unit Delay With Preview Enabled Resettable External RV/1 -> Xnew/1
  IV/1 -> Unit Delay With Preview Enabled Resettable External RV/4
  R/1 -> Unit Delay With Preview Enabled Resettable External RV/3
  E/1 -> Unit Delay With Preview Enabled Resettable External RV/2
  Xcalc/1 -> Unit Delay With Preview Enabled Resettable External RV/1

== system fixpt_megmalib/Counters and Timers/Timer RetriggerResetEnabled/ResetEnabledState ==
  E : Inport  LatchInput=off
  R : Inport  Port=2  LatchInput=off
  IV : Inport  Port=3  LatchInput=off
  Xcalc : Inport  Port=4  LatchInput=off
  Unit Delay With Preview Enabled Resettable External RV : simulink/Additional Math & Discrete/Additional Discrete/Unit Delay With Preview Enabled Resettable External RV  vinit=0.0  tsamp=-1
  Xnew : Outport
  Xold : Outport  Port=2
  wires:
  Unit Delay With Preview Enabled Resettable External RV/2 -> Xold/1
  Unit Delay With Preview Enabled Resettable External RV/1 -> Xnew/1
  IV/1 -> Unit Delay With Preview Enabled Resettable External RV/4
  R/1 -> Unit Delay With Preview Enabled Resettable External RV/3
  E/1 -> Unit Delay With Preview Enabled Resettable External RV/2
  Xcalc/1 -> Unit Delay With Preview Enabled Resettable External RV/1

== system fixpt_megmalib/Integrators/Accumulator/ResetEnabledState ==
  E : Inport  LatchInput=off
  R : Inport  Port=2  LatchInput=off
  IV : Inport  Port=3  LatchInput=off
  Xcalc : Inport  Port=4  LatchInput=off
  Unit Delay With Preview Enabled Resettable External RV : simulink/Additional Math & Discrete/Additional Discrete/Unit Delay With Preview Enabled Resettable External RV  vinit=0.0  tsamp=-1
  Xnew : Outport
  Xold : Outport  Port=2
  wires:
  Unit Delay With Preview Enabled Resettable External RV/2 -> Xold/1
  Unit Delay With Preview Enabled Resettable External RV/1 -> Xnew/1
  IV/1 -> Unit Delay With Preview Enabled Resettable External RV/4
  R/1 -> Unit Delay With Preview Enabled Resettable External RV/3
  E/1 -> Unit Delay With Preview Enabled Resettable External RV/2
  Xcalc/1 -> Unit Delay With Preview Enabled Resettable External RV/1

== system fixpt_megmalib/Low and Highpass/DigitalLowPass ResetEnabled/ResetEnabledState ==
  E : Inport  LatchInput=off
  R : Inport  Port=2  LatchInput=off
  IV : Inport  Port=3  LatchInput=off
  Xcalc : Inport  Port=4  LatchInput=off
  Unit Delay With Preview Enabled Resettable External RV : simulink/Additional Math & Discrete/Additional Discrete/Unit Delay With Preview Enabled Resettable External RV  vinit=0.0  tsamp=-1
  Xnew : Outport
  Xold : Outport  Port=2
  wires:
  Unit Delay With Preview Enabled Resettable External RV/2 -> Xold/1
  Unit Delay With Preview Enabled Resettable External RV/1 -> Xnew/1
  IV/1 -> Unit Delay With Preview Enabled Resettable External RV/4
  R/1 -> Unit Delay With Preview Enabled Resettable External RV/3
  E/1 -> Unit Delay With Preview Enabled Resettable External RV/2
  Xcalc/1 -> Unit Delay With Preview Enabled Resettable External RV/1

== system fixpt_megmalib/Low and Highpass/HighPass TResetEnabled/ResetEnabledState ==
  E : Inport  LatchInput=off
  R : Inport  Port=2  LatchInput=off
  IV : Inport  Port=3  LatchInput=off
  Xcalc : Inport  Port=4  LatchInput=off
  Unit Delay With Preview Enabled Resettable External RV : simulink/Additional Math & Discrete/Additional Discrete/Unit Delay With Preview Enabled Resettable External RV  vinit=0.0  tsamp=-1
  Xnew : Outport
  Xold : Outport  Port=2
  wires:
  Unit Delay With Preview Enabled Resettable External RV/2 -> Xold/1
  Unit Delay With Preview Enabled Resettable External RV/1 -> Xnew/1
  IV/1 -> Unit Delay With Preview Enabled Resettable External RV/4
  R/1 -> Unit Delay With Preview Enabled Resettable External RV/3
  E/1 -> Unit Delay With Preview Enabled Resettable External RV/2
  Xcalc/1 -> Unit Delay With Preview Enabled Resettable External RV/1

== system fixpt_megmalib/Low and Highpass/LowPass KResetEnabled/ResetEnabledState ==
  E : Inport  LatchInput=off
  R : Inport  Port=2  LatchInput=off
  IV : Inport  Port=3  LatchInput=off
  Xcalc : Inport  Port=4  LatchInput=off
  Unit Delay With Preview Enabled Resettable External RV : simulink/Additional Math & Discrete/Additional Discrete/Unit Delay With Preview Enabled Resettable External RV  vinit=0.0  tsamp=-1
  Xnew : Outport
  Xold : Outport  Port=2
  wires:
  Unit Delay With Preview Enabled Resettable External RV/2 -> Xold/1
  Unit Delay With Preview Enabled Resettable External RV/1 -> Xnew/1
  IV/1 -> Unit Delay With Preview Enabled Resettable External RV/4
  R/1 -> Unit Delay With Preview Enabled Resettable External RV/3
  E/1 -> Unit Delay With Preview Enabled Resettable External RV/2
  Xcalc/1 -> Unit Delay With Preview Enabled Resettable External RV/1
